simulink model "GRM_Airframe"  (R2018b)
settings: Solver=FixedStepAuto  StartTime=0.0  StopTime=T_sim  FixedStep=0.001  RelTol=1e-3
PreLoadFcn:
  | addpath('init_functions');
  | init_grm;
  | addpath('parameters');
  | para_def_grm;
values from neighbouring files (symbols this model uses):
  act_dmp = 0.6322    [para_def_grm.m]
  act_omega = 59.9250    (= 59.925)    [para_def_grm.m]
  aero = load('aero.mat')    [para_def_grm.m]
  c_be = -6.5e-3    (= -0.0065)    [init_grm.m]
  c_h_geop0 = 0    [init_grm.m]
  c_h_geope = 11e3    (= 11000)    [init_grm.m]
  c_pa0 = 101325    [init_grm.m]
  c_pe = -c_g0/c_be/sgc    (= 5.25587981272)    [init_grm.m]
  c_r0 = 6371000.79    [init_grm.m]
  c_rot = 7.292115e-5    (= 7.292115e-05)    [init_grm.m]
  c_Tmp0 = 288.15    [init_grm.m]
  d_siB_0 = 0    [para_def_grm.m]
  d_siB_max = deg2rad(1200)    [para_def_grm.m]
  d_siB_min = deg2rad(-1200)    [para_def_grm.m]
  dd_siB_max = deg2rad(50000)    [para_def_grm.m]
  dd_siB_min = deg2rad(-50000)    [para_def_grm.m]
  de_JBBB_xx = JBBB_xx_0 - JBBB_xx_e    (= 0)    [para_def_grm.m]
  de_JBBB_yy = JBBB_yy_0 - JBBB_yy_e    (= 0)    [para_def_grm.m]
  de_JBBB_zz = JBBB_zz_0 - JBBB_zz_e    (= 0)    [para_def_grm.m]
  de_mM = m_fuel_lookup(end)    [para_def_grm.m]
  F_prp = [450.52;428.7;423.25;391.61;352.34;304.35;266.17;243.26;216.92 ... (first row only)    [para_def_grm.m]
  flag_I_aero_switch = 1    [init_grm.m]
  flag_I_flat = 1    [init_grm.m]
  flag_I_gravity_switch = 1    [init_grm.m]
  flag_I_rot = 0    [init_grm.m]
  hcr = 1.4    [init_grm.m]
  J0PB_e = TBP*J0PP_e*TBP'    [para_def_grm.m]
  JMMM_0 = TBP*J0PP_0*TBP'    [para_def_grm.m]
  JMMM_e = TBP*J0PP_e*TBP'    [para_def_grm.m]
  lat_0 = 0    [init_grm.m]
  lon_0 = 0    [init_grm.m]
  m0 = mB_0    (= 3.30977)    [para_def_grm.m]
  m_fuel_lookup = [0;0.0573;0.1127;0.1667;0.2186;0.2681;0.3149;0.3588 ... (first row only)    [para_def_grm.m]
  mB_0 = 3.30977    [para_def_grm.m]
  mM_0 = 1.119    [para_def_grm.m]
  mM_e = de_mM    [para_def_grm.m]
  p0PB = [x0PB;y0PB;z0PB]    [para_def_grm.m]
  pBII_0 = TIE_0*pBEE_0    [init_grm.m]
  pMPB = [xMPB;yMPB;zMPB]    [para_def_grm.m]
  pNPB = [0;0;0]    [para_def_grm.m]
  qEG_0 = q12_from_T12(TEG)    [init_grm.m]
  qIB_0 = qumul(qIG_0,qGB_0)    [init_grm.m]
  qIE_0 = q12_from_T12(TIE_0)    [init_grm.m]
  sgc = 287.05287    [init_grm.m]
  siB_0 = 0    [para_def_grm.m]
  siB_max = deg2rad(30)    [para_def_grm.m]
  siB_min = deg2rad(-30)    [para_def_grm.m]
  t_prp1 = [0.04;0.28;0.54;1;1.48;1.99;2.51;3;3.5;3.67;3.82;4]    [para_def_grm.m]
  t_prp2 = t_prp2'    [para_def_grm.m]
  Tr3r4 = [1,1,1,1;1,1,-1,-1;-1,1,1,-1]*0.25    [para_def_grm.m]
  tRRR = 0    [para_def_grm.m]
  unc_act_bl = 0    [para_def_grm.m]
  unc_act_off = 0    [para_def_grm.m]
  unc_act_scale = 1    [para_def_grm.m]
  unc_aero_Cl_scale = 1    [para_def_grm.m]
  unc_aero_Cm_scale = 1    [para_def_grm.m]
  unc_aero_Cn_scale = 1    [para_def_grm.m]
  unc_aero_Cx_scale = 1    [para_def_grm.m]
  unc_aero_Cy_scale = 1    [para_def_grm.m]
  unc_aero_Cz_scale = 1    [para_def_grm.m]
  unc_cg_x = 0    [para_def_grm.m]
  unc_cg_y = 0    [para_def_grm.m]
  unc_cg_z = 0    [para_def_grm.m]
  unc_mB_bl = 0    [para_def_grm.m]
  unc_mB_scale = 1    [para_def_grm.m]
  unc_moi_Jxx = 0    [para_def_grm.m]
  unc_moi_Jyy = 0    [para_def_grm.m]
  unc_moi_Jzz = 0    [para_def_grm.m]
  unc_prp_scale = 1    [para_def_grm.m]
  unc_prp_x = 0    [para_def_grm.m]
  unc_prp_y = 0    [para_def_grm.m]
  unc_prp_z = 0    [para_def_grm.m]
  vBII_0 = vBEE_0 + cross(wIEI_0,pBII_0)    [init_grm.m]
  wBIB_0 = r2_from_r1_trans_q21(wBII_0,qBI_0)    [init_grm.m]
  x0PB = -0.5    [para_def_grm.m]
  xMPB = -0.9    [para_def_grm.m]
  y0PB = 0    [para_def_grm.m]
  yMPB = 0    [para_def_grm.m]
  z0PB = 0    [para_def_grm.m]
  zMPB = 0    [para_def_grm.m]
undefined symbols (not defined in the file or in its folder): c_b_WGS, c_flat, c_grav, c_rsma, d_mB_lookup, t_dmB
libraries: simulink_extras x11, simulink x3
(part 2 of 6)

== system GRM_Airframe/GRM_Airframe/weight_and_balance/d_moi ==
  prp : Inport
  Bus Selector1 : BusSelector  OutputSignals=dmB
  Constant : Constant  Value=de_JBBB_zz
  Constant1 : Constant  Value=de_JBBB_xx
  Constant2 : Constant  Value=de_JBBB_yy
  Constant5 : Constant  Value=de_mM
  Divide : Product  Inputs=*/
  Divide1 : Product  Inputs=*/
  Divide2 : Product  Inputs=*/
  Product : Product
  Vector Concatenate : Concatenate  NumInputs=3
  vector2diagonal_matrix : Subsystem
  d_JBBB : Outport
  wires:
  Constant2/1 -> Divide1/1
  prp/1 -> Bus Selector1/1
  Vector Concatenate/1 -> vector2diagonal_matrix/1(vector)
  Constant1/1 -> Divide2/1
  Divide/1 -> Vector Concatenate/3
  Divide1/1 -> Vector Concatenate/2
  Constant/1 -> Divide/1
  Constant5/1 -> Divide/2, Divide1/2, Divide2/2
  Divide2/1 -> Vector Concatenate/1
  Bus Selector1/1 -> Product/2  "<dmB>"
  vector2diagonal_matrix/1(diagonal_matrix) -> Product/1
  Product/1 -> d_JBBB/1  "d_JBBB"

== system GRM_Airframe/GRM_Airframe/weight_and_balance/mass ==
  sim_time_launch : Inport
  1-D Lookup Table : Lookup_n-D  NumberOfTableDimensions=1  BreakpointsForDimension1=t_prp2  Table=m_fuel_lookup  ExtrapMethod=Clip  DiagnosticForOutOfRangeInput=Warning  UseLastTableValue=on  InternalRulePriority=Speed  RndMeth=Simplest  InputSameDT=on
  Add : Sum  Inputs=+-
  Constant : Constant  Value=0
  Constant1 : Constant  Value=mB_0
  Constant2 : Constant  Value=mM_0
  Saturation : Saturate  UpperLimit=t_prp2(end)  LowerLimit=0
      settings: AttributesFormatString=|
      | %<UpperLimit>
      | %<LowerLimit>
  Subtract1 : Sum  Inputs=+-+
  Switch : Switch  Criteria=u2 > Threshold
  Switch1 : Switch  Criteria=u2 > Threshold
  mB_c : Outport
  mM : Outport  Port=2
  wires:
  Add/1 -> mM/1  "mM"
  Constant2/1 -> Add/1, Subtract1/3
  Saturation/1 -> 1-D Lookup Table/1
  sim_time_launch/1 -> Switch/2, Switch/1
  Constant/1 -> Switch/3
  1-D Lookup Table/1 -> Switch1/1
  Switch/1 -> Switch1/3, Switch1/2, Saturation/1
  Subtract1/1 -> mB_c/1  "mB_c"
  Switch1/1 -> Subtract1/2, Add/2
  Constant1/1 -> Subtract1/1

== system GRM_Airframe/GRM_Airframe/weight_and_balance/mass_uncertainty ==
  mB_c : Inport
  Add : Sum
  Constant : Constant  Value=unc_mB_bl
  Constant1 : Constant  Value=unc_mB_scale
  Product : Product
  mB : Outport
  wires:
  Product/1 -> Add/2
  Constant1/1 -> Product/2
  Add/1 -> mB/1  "mB"
  mB_c/1 -> Product/1
  Constant/1 -> Add/1

== system GRM_Airframe/GRM_Airframe/weight_and_balance/moi ==
  pBPB : Inport
  mM : Inport  Port=2
  Add : Sum
  Add4 : Sum
  Add5 : Sum
  Constant15 : Constant  Value=J0PB_e
  JMMM_linear_interpolation : Subsystem
  moi_coordinate_transformation : Subsystem
  moi_uncertainty : Subsystem
  steiners_theorem_missile : Subsystem
  steiners_theorem_motor : Subsystem
  JBBB : Outport
  wires:
  moi_uncertainty/1(JBBB) -> JBBB/1
  Add4/1 -> moi_uncertainty/1(JBBB_c)  "JBBB_c"
  steiners_theorem_missile/1(J_deviation) -> Add5/2
  Add5/1 -> Add4/1  "J0BB"
  Constant15/1 -> Add5/1
  Add/1 -> Add4/2  "JMBB"
  steiners_theorem_motor/1(JM_deviation) -> Add/1
  pBPB/1 -> steiners_theorem_motor/1(pBPB), steiners_theorem_missile/1(pBPB)
  moi_coordinate_transformation/1(JMMB) -> Add/2
  JMMM_linear_interpolation/1(JMMM) -> moi_coordinate_transformation/1(JMMM)
  mM/1 -> JMMM_linear_interpolation/1(mM), steiners_theorem_motor/2(mM)

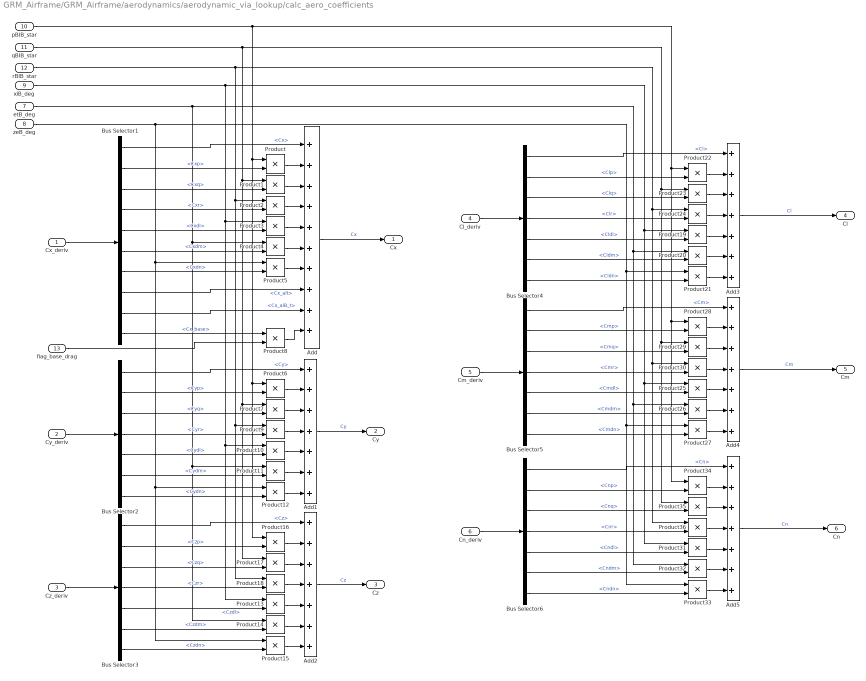
== system GRM_Airframe/GRM_Airframe/aerodynamics/aerodynamic_via_lookup/calc_aero_coefficients ==
  Cx_deriv : Inport
  Cy_deriv : Inport  Port=2
  Cz_deriv : Inport  Port=3
  Cl_deriv : Inport  Port=4
  Cm_deriv : Inport  Port=5
  Cn_deriv : Inport  Port=6
  etB_deg : Inport  Port=7
  zeB_deg : Inport  Port=8
  xiB_deg : Inport  Port=9
  pBIB_star : Inport  Port=10
  qBIB_star : Inport  Port=11
  rBIB_star : Inport  Port=12
  flag_base_drag : Inport  Port=13
  Add : Sum  Inputs=++++++++++
  Add{1..5} (5 alike) : Sum  Inputs=+++++++
  Bus Selector1 : BusSelector  OutputSignals=Cx,Cxp,Cxq,Cxr,Cxdl,Cxdm,Cxdn,Cx_alt,Cx_alB_t,Cx_base
  Bus Selector2 : BusSelector  OutputSignals=Cy,Cyp,Cyq,Cyr,Cydl,Cydm,Cydn
  Bus Selector3 : BusSelector  OutputSignals=Cz,Czp,Czq,Czr,Czdl,Czdm,Czdn
  Bus Selector4 : BusSelector  OutputSignals=Cl,Clp,Clq,Clr,Cldl,Cldm,Cldn
  Bus Selector5 : BusSelector  OutputSignals=Cm,Cmp,Cmq,Cmr,Cmdl,Cmdm,Cmdn
  Bus Selector6 : BusSelector  OutputSignals=Cn,Cnp,Cnq,Cnr,Cndl,Cndm,Cndn
  Product{,1..36} (37 alike) : Product
  Cx : Outport
  Cy : Outport  Port=2
  Cz : Outport  Port=3
  Cl : Outport  Port=4
  Cm : Outport  Port=5
  Cn : Outport  Port=6
  wires:
  zeB_deg/1 -> Product5/1, Product12/1, Product15/1, Product21/1, Product33/1, Product27/1
  Bus Selector6/1 -> Add5/1  "<Cn>"
  Bus Selector6/7 -> Product33/2  "<Cndn>"
  Bus Selector6/6 -> Product32/2  "<Cndm>"
  Bus Selector6/5 -> Product31/2  "<Cndl>"
  Bus Selector6/4 -> Product36/2  "<Cnr>"
  Bus Selector6/3 -> Product35/2  "<Cnq>"
  Bus Selector6/2 -> Product34/2  "<Cnp>"
  Add5/1 -> Cn/1  "Cn"
  Product33/1 -> Add5/7
  Product32/1 -> Add5/6
  Product31/1 -> Add5/5
  Product36/1 -> Add5/4
  Product35/1 -> Add5/3
  Product34/1 -> Add5/2
  Bus Selector5/7 -> Product27/2  "<Cmdn>"
  Bus Selector5/6 -> Product26/2  "<Cmdm>"
  Bus Selector5/5 -> Product25/2  "<Cmdl>"
  Bus Selector5/4 -> Product30/2  "<Cmr>"
  Bus Selector5/3 -> Product29/2  "<Cmq>"
  Bus Selector5/2 -> Product28/2  "<Cmp>"
  Bus Selector5/1 -> Add4/1  "<Cm>"
  Add4/1 -> Cm/1  "Cm"
  Product27/1 -> Add4/7
  Product26/1 -> Add4/6
  Product25/1 -> Add4/5
  Product30/1 -> Add4/4
  Product29/1 -> Add4/3
  Product28/1 -> Add4/2
  Bus Selector4/1 -> Add3/1  "<Cl>"
  Bus Selector4/7 -> Product21/2  "<Cldn>"
  Bus Selector4/6 -> Product20/2  "<Cldm>"
  Bus Selector4/5 -> Product19/2  "<Cldl>"
  Bus Selector4/4 -> Product24/2  "<Clr>"
  Bus Selector4/3 -> Product23/2  "<Clq>"
  Bus Selector4/2 -> Product22/2  "<Clp>"
  Add3/1 -> Cl/1  "Cl"
  Product21/1 -> Add3/7
  Product20/1 -> Add3/6
  Product19/1 -> Add3/5
  Product24/1 -> Add3/4
  Product23/1 -> Add3/3
  Product22/1 -> Add3/2
  Bus Selector3/7 -> Product15/2  "<Czdn>"
  Bus Selector3/6 -> Product14/2  "<Czdm>"
  Bus Selector3/5 -> Product13/2  "<Czdl>"
  Bus Selector3/4 -> Product18/2  "<Czr>"
  Bus Selector3/3 -> Product17/2  "<Czq>"
  Bus Selector3/1 -> Add2/1  "<Cz>"
  Bus Selector3/2 -> Product16/2  "<Czp>"
  Add2/1 -> Cz/1  "Cz"
  Product15/1 -> Add2/7
  Product14/1 -> Add2/6
  Product13/1 -> Add2/5
  Product18/1 -> Add2/4
  Product17/1 -> Add2/3
  Product16/1 -> Add2/2
  Add1/1 -> Cy/1  "Cy"
  Add/1 -> Cx/1  "Cx"
  rBIB_star/1 -> Product2/1, Product9/1, Product18/1, Product24/1, Product30/1, Product36/1
  qBIB_star/1 -> Product1/1, Product7/1, Product17/1, Product23/1, Product29/1, Product35/1
  pBIB_star/1 -> Product/1, Product6/1, Product16/1, Product22/1, Product28/1, Product34/1
  Bus Selector2/7 -> Product12/2  "<Cydn>"
  Bus Selector2/6 -> Product11/2  "<Cydm>"
  Bus Selector2/5 -> Product10/2  "<Cydl>"
  Bus Selector2/4 -> Product9/2  "<Cyr>"
  Bus Selector2/3 -> Product7/2  "<Cyq>"
  Product12/1 -> Add1/7
  Product11/1 -> Add1/6
  Product10/1 -> Add1/5
  Product9/1 -> Add1/4
  Product7/1 -> Add1/3
  Bus Selector2/2 -> Product6/2  "<Cyp>"
  Product6/1 -> Add1/2
  Bus Selector2/1 -> Add1/1  "<Cy>"
  etB_deg/1 -> Product4/1, Product11/1, Product14/1, Product20/1, Product26/1, Product32/1
  xiB_deg/1 -> Product3/1, Product10/1, Product13/1, Product19/1, Product25/1, Product31/1
  flag_base_drag/1 -> Product8/2
  Bus Selector1/10 -> Product8/1  "<Cx_base>"
  Product8/1 -> Add/10
  Bus Selector1/9 -> Add/9  "<Cx_alB_t>"
  Bus Selector1/8 -> Add/8  "<Cx_alt>"
  Product5/1 -> Add/7
  Bus Selector1/7 -> Product5/2  "<Cxdn>"
  Product4/1 -> Add/6
  Bus Selector1/6 -> Product4/2  "<Cxdm>"
  Product3/1 -> Add/5
  Bus Selector1/5 -> Product3/2  "<Cxdl>"
  Product2/1 -> Add/4
  Bus Selector1/4 -> Product2/2  "<Cxr>"
  Bus Selector1/3 -> Product1/2  "<Cxq>"
  Product1/1 -> Add/3
  Product/1 -> Add/2
  Bus Selector1/2 -> Product/2  "<Cxp>"
  Bus Selector1/1 -> Add/1  "<Cx>"
  Cl_deriv/1 -> Bus Selector4/1
  Cz_deriv/1 -> Bus Selector3/1
  Cm_deriv/1 -> Bus Selector5/1
  Cn_deriv/1 -> Bus Selector6/1
  Cy_deriv/1 -> Bus Selector2/1
  Cx_deriv/1 -> Bus Selector1/1

== system GRM_Airframe/GRM_Airframe/aerodynamics/aerodynamic_via_lookup/calc_aero_for_mom ==
  hBE : Inport
  pBSB : Inport  Port=2
  qdynB : Inport  Port=3
  Cx : Inport  Port=4
  Cy : Inport  Port=5
  Cz : Inport  Port=6
  Cl : Inport  Port=7
  Cm : Inport  Port=8
  Cn : Inport  Port=9
  Add : Sum
  Constant1 : Constant  Value=aero.lref
  Constant2 : Constant  Value=aero.sref
  Product : Product
  Product1 : Product  Inputs=3
  Product2 : Product
  Vector Concatenate1 : Concatenate  NumInputs=3
  Vector Concatenate2 : Concatenate  NumInputs=3
  cross_product : Subsystem
      mask help: cross product r3 = r1 x r2
      mask Help:
      | Name:
      | 
      |     cross_product
      | 
      | Description:
      | 
      |     This block implements the cross product r3 = r1 x r2.
      | 
      | Inputs  [size] [data type] [unit]:
      | 
      |     vector 1  [3] [double] [-]
      |     vector 2  [3] [double] [-]
      | 
      | Outputs  [size] [data type] [unit]:
      | 
      |     resulting vector  [3] [double] [-]
      mask Display: disp(' r3 = r1 x r2')
  launch_rail : Subsystem
  launch_rail1 : Subsystem
  FBAB : Outport
  MBAB : Outport  Port=2
  wires:
  launch_rail/1(FBAB) -> FBAB/1
  launch_rail1/1(MBAB) -> MBAB/1
  hBE/1 -> launch_rail/1(hBE), launch_rail1/1(hBE)
  cross_product/1(r1_x_r2) -> Add/1
  Product2/1 -> Product/2, Product1/1
  Constant2/1 -> Product2/1
  Constant1/1 -> Product1/3
  Add/1 -> launch_rail1/2(MBAB_c)  "MBAB"
  Product1/1 -> Add/2  "MBAB"
  Product/1 -> cross_product/2(r2), launch_rail/2(FBAB_c)  "FBAB"
  pBSB/1 -> cross_product/1(r1)
  Vector Concatenate2/1 -> Product/1
  Vector Concatenate1/1 -> Product1/2
  qdynB/1 -> Product2/2
  Cn/1 -> Vector Concatenate1/3
  Cl/1 -> Vector Concatenate1/1
  Cx/1 -> Vector Concatenate2/1
  Cz/1 -> Vector Concatenate2/3
  Cm/1 -> Vector Concatenate1/2
  Cy/1 -> Vector Concatenate2/2

== system GRM_Airframe/GRM_Airframe/aerodynamics/aerodynamic_via_lookup/calc_derivatives ==
  hBE : Inport
  MaB : Inport  Port=2
  alB : Inport  Port=3
  beB : Inport  Port=4
  etB_deg : Inport  Port=5
  zeB_deg : Inport  Port=6
  Cl_derivatives_lookup : Subsystem
  Cm_derivatives_lookup : Subsystem
  Cn_derivatives_lookup : Subsystem
  Cx_derivatives_lookup : Subsystem
  Cy_derivatives_lookup : Subsystem
  Cz_derivatives_lookup : Subsystem
  aerodynamics_pre_lookup : Subsystem
  calc_total_deflection_angle : Subsystem
  Cx_deriv : Outport
  Cy_deriv : Outport  Port=2
  Cz_deriv : Outport  Port=3
  Cl_deriv : Outport  Port=4
  Cm_deriv : Outport  Port=5
  Cn_deriv : Outport  Port=6
  wires:
  zeB_deg/1 -> calc_total_deflection_angle/2(zeB_deg)
  etB_deg/1 -> calc_total_deflection_angle/1(etB_deg)
  beB/1 -> aerodynamics_pre_lookup/2(beB), calc_total_deflection_angle/4(beB)
  alB/1 -> aerodynamics_pre_lookup/1(alB), calc_total_deflection_angle/3(alB)
  calc_total_deflection_angle/1(delta_t) -> Cx_derivatives_lookup/1(delta_t)
  hBE/1 -> Cx_derivatives_lookup/2(hBE)
  aerodynamics_pre_lookup/1(aero_pre_lookup) -> Cx_derivatives_lookup/3(aero_pre_lookup), Cy_derivatives_lookup/1(aero_pre_lookup), Cz_derivatives_lookup/1(aero_pre_lookup), Cl_derivatives_lookup/1(aero_pre_lookup), Cm_derivatives_lookup/1(aero_pre_lookup), Cn_derivatives_lookup/1(aero_pre_lookup)
  Cl_derivatives_lookup/1(Cl_deriv) -> Cl_deriv/1
  Cm_derivatives_lookup/1(Cm_deriv) -> Cm_deriv/1
  Cz_derivatives_lookup/1(Cz_deriv) -> Cz_deriv/1
  Cy_derivatives_lookup/1(Cy_deriv) -> Cy_deriv/1
  MaB/1 -> aerodynamics_pre_lookup/3(Ma)
  Cx_derivatives_lookup/1(Cx_deriv) -> Cx_deriv/1
  Cn_derivatives_lookup/1(Cn_deriv) -> Cn_deriv/1

== system GRM_Airframe/GRM_Airframe/aerodynamics/aerodynamic_via_lookup/transform_rad2deg_al_be ==
  alB : Inport
  beB : Inport  Port=2
  Radians to Degrees : simulink_extras/Transformations/Radians to Degrees
  Radians to Degrees1 : simulink_extras/Transformations/Radians to Degrees
  alB_deg : Outport
  beB_deg : Outport  Port=2
  wires:
  beB/1 -> Radians to Degrees1/1
  Radians to Degrees1/1 -> beB_deg/1  "beB_deg"
  Radians to Degrees/1 -> alB_deg/1  "alB_deg"
  alB/1 -> Radians to Degrees/1

== system GRM_Airframe/GRM_Airframe/aerodynamics/aerodynamic_via_lookup/transform_rad2deg_fin ==
  afinB : Inport
  Demux : Demux  Outputs=3
  Radians to Degrees : simulink_extras/Transformations/Radians to Degrees
  Radians to Degrees1 : simulink_extras/Transformations/Radians to Degrees
  Radians to Degrees2 : simulink_extras/Transformations/Radians to Degrees
  etB_deg : Outport
  zeB_deg : Outport  Port=2
  xiB_deg : Outport  Port=3
  wires:
  Demux/1 -> Radians to Degrees/1  "xiB"
  afinB/1 -> Demux/1
  Demux/3 -> Radians to Degrees2/1  "zeB"
  Demux/2 -> Radians to Degrees1/1  "etB"
  Radians to Degrees1/1 -> etB_deg/1  "etB_deg"
  Radians to Degrees2/1 -> zeB_deg/1  "zeB_deg"
  Radians to Degrees/1 -> xiB_deg/1  "xiB_deg"

== system GRM_Airframe/GRM_Airframe/aerodynamics/aerodynamic_via_lookup/transform_rad2deg_rates ==
  wBIB_star : Inport
  Demux : Demux  Outputs=3
  Radians to Degrees : simulink_extras/Transformations/Radians to Degrees
  Radians to Degrees1 : simulink_extras/Transformations/Radians to Degrees
  Radians to Degrees2 : simulink_extras/Transformations/Radians to Degrees
  pBIB_star_deg : Outport
  qBIB_star_deg : Outport  Port=2
  rBIB_star_deg : Outport  Port=3
  wires:
  Radians to Degrees1/1 -> qBIB_star_deg/1  "qBIB_star_deg"
  Demux/2 -> Radians to Degrees1/1
  Radians to Degrees/1 -> pBIB_star_deg/1  "pBIB_star_deg"
  Demux/1 -> Radians to Degrees/1
  wBIB_star/1 -> Demux/1
  Radians to Degrees2/1 -> rBIB_star_deg/1  "rBIB_star_deg"
  Demux/3 -> Radians to Degrees2/1

== system GRM_Airframe/GRM_Airframe/environment/WGS84_Gravitation/WGS84_2_ECEF ==
  h : Inport
  lon : Inport  Port=2
  lat : Inport  Port=3
  Add1 : Sum  Inputs=+-
  Add2 : Sum
  Add3 : Sum
  Constant : Constant
  Divide : Product  Inputs=***
  Divide1 : Product  Inputs=***
  Divide2 : Product  Inputs=**
  Divide3 : Product  Inputs=**
  Divide4 : Product  Inputs=**
  Mux : Mux  Inputs=3
  Trigonometric Function : Trigonometry
  Trigonometric Function1 : Trigonometry  Operator=cos
  Trigonometric Function2 : Trigonometry
  Trigonometric Function3 : Trigonometry  Operator=cos
  "WGS84 Transformation Parameter " : Subsystem
  pE : Outport
  wires:
  Trigonometric Function/1 -> Divide1/2  "sin(lambda)"
  Trigonometric Function2/1 -> Divide4/2  "sin(phi)"
  Add3/1 -> Divide/1, Divide1/1
  lon/1 -> Trigonometric Function/1, Trigonometric Function1/1
  Mux/1 -> pE/1  "pE"
  Trigonometric Function3/1 -> Divide/3, Divide1/3  "cos(phi)"
  Trigonometric Function1/1 -> Divide/2  "cos(lambda)"
  h/1 -> Add3/1, Add2/1
  "WGS84 Transformation Parameter "/2(e) -> Divide2/1, Divide2/2
  "WGS84 Transformation Parameter "/1(N) -> Divide3/1, Add3/2
  Divide4/1 -> Mux/3  "z_ECEF"
  Add1/1 -> Divide3/2
  Constant/1 -> Add1/1
  Divide3/1 -> Add2/2  "N(1-e^2)"
  Divide2/1 -> Add1/2
  lat/1 -> Trigonometric Function2/1, Trigonometric Function3/1, "WGS84 Transformation Parameter "/1(phi)
  Divide/1 -> Mux/1  "x_ECEF"
  Add2/1 -> Divide4/1
  Divide1/1 -> Mux/2  "y_ECEF"

== system GRM_Airframe/GRM_Airframe/environment/atmosphere_static_ISO_2533/density ==
  Tmp : Inport
  pa : Inport  Port=2
  Divide : Product  Inputs=/*/
  specific_gas_constant : Constant  Value=sgc
  rho : Outport
  wires:
  specific_gas_constant/1 -> Divide/3
  pa/1 -> Divide/2
  Divide/1 -> rho/1  "rho"
  Tmp/1 -> Divide/1

== system GRM_Airframe/GRM_Airframe/environment/atmosphere_static_ISO_2533/geopot_height ==
  hBE : Inport
  Add : Sum
  Divide : Product  Inputs=*/*
  mean_earth_radius : Constant  Value=mean_earth_radius
  h_geop : Outport
  wires:
  Add/1 -> Divide/2
  hBE/1 -> Divide/1, Add/1
  Divide/1 -> h_geop/1  "h_geop"
  mean_earth_radius/1 -> Add/2, Divide/3

== system GRM_Airframe/GRM_Airframe/environment/atmosphere_static_ISO_2533/speed_of_sound ==
  Tmp : Inport
  Product : Product  Inputs=3
  Sqrt : Sqrt  SaturateOnIntegerOverflow=on
  heat_capacity_ratio : Constant  Value=hcr
  specific_gas_constant : Constant  Value=sgc
  sos : Outport
  wires:
  specific_gas_constant/1 -> Product/1
  heat_capacity_ratio/1 -> Product/2
  Product/1 -> Sqrt/1
  Tmp/1 -> Product/3
  Sqrt/1 -> sos/1  "sos"

== system GRM_Airframe/GRM_Airframe/environment/atmosphere_static_ISO_2533/tmp_and_pressure_ISO_2533 ==
  h_geop : Inport
  e_Tmp : Inport  Port=2
  e_pa : Inport  Port=3
  Subtract1 : Sum
  Subtract2 : Sum
  Tmp_norm_msl : Constant  Value=c_Tmp0
  geopotential_height_ref : Constant  Value=c_h_geop0
  pa_norm_msl : Constant  Value=c_pa0
  static_Temperature : Subsystem
  static_pressure : Subsystem
  Tmp : Outport
  pa : Outport  Port=2
  wires:
  Tmp_norm_msl/1 -> Subtract1/2
  geopotential_height_ref/1 -> static_Temperature/3(h_geop_ref), static_pressure/1(h_geop_ref)  "h_geop_ref"
  e_Tmp/1 -> Subtract1/1
  static_Temperature/1(Tmp) -> Tmp/1
  e_pa/1 -> Subtract2/1
  static_pressure/1(pa) -> pa/1
  Subtract1/1 -> static_Temperature/1(Tmp_ref), static_pressure/3(Tmp_ref)  "Tmp_ref"
  pa_norm_msl/1 -> Subtract2/2
  Subtract2/1 -> static_pressure/4(pa_ref)  "pa_ref"
  h_geop/1 -> static_Temperature/2(h_geop), static_pressure/2(h_geop)

== system GRM_Airframe/GRM_Airframe/gravity/launch_rail/initial_altitude ==
  Constant : Constant  Value=pBII_0
  Constant2 : Constant  Value=flag_I_flat
  Demux : Demux  Outputs=3
  Gain : Gain  Gain=-1
  Switch1 : Switch  Criteria=u2 > Threshold
  Terminator{,1..3} (4 alike) : Terminator
  trafo_E_to_geodetic : Subsystem  mask(Transformation der ECEF Position in geodätische Größen){}
      mask help: Dieser Block transformiert die Position im ECEF KOS in die geodätische Länge, Breite und Höhe
      mask init:
      | [c_mue, c_rsma, c_flat] = init_transformations_earth;
      mask Help:
      | Name:
      | 
      |     trafo_E_to_geodetic
      | 
      | Beschreibung:
      | 
      |     Dieser Block transformiert die Position im ECEF KOS in die geodätische
      |     Länge, Breite und Höhe.
      | 
      | Inputs   [size]  [data type] [unit]:
      | 
      |     pBEE    [3] [double] [m]
      | 
      | Outputs  [size]  [data type] [unit]:
      | 
      |     long  [1] [double] [rad]
      |     lat   [1] [double] [rad]
      |     alt   [1] [double] [m]
      | 
      | Parameter
      | 
      |    c_rsma
      |    c_flat
  hBE_0 : Outport
  wires:
  Switch1/1 -> hBE_0/1  "hBE_0"
  trafo_E_to_geodetic/1(lon) -> Terminator/1
  Constant/1 -> trafo_E_to_geodetic/1(pBEE), Demux/1
  trafo_E_to_geodetic/2(lat) -> Terminator1/1
  Demux/1 -> Terminator2/1
  Gain/1 -> Switch1/1
  Demux/3 -> Gain/1
  Demux/2 -> Terminator3/1
  trafo_E_to_geodetic/3(alt) -> Switch1/3  "hBE_0"
  Constant2/1 -> Switch1/2

== system GRM_Airframe/GRM_Airframe/motion_kinematics/calc_motion_kinematics/calc_transformation_matrix ==
  qIE : Inport
  qEG : Inport  Port=2
  qIB : Inport  Port=3
  T12_from_q1 : Subsystem
      mask help: Transforms a quaternion into a Direction Cosine Matrix
      mask Help:
      | Name:
      | 
      |     T12_from_q12
      | 
      | Description:
      | 
      |     This block implements the transformation of a quaternion into the
      |     corresponding direction cosine matrix DCM.
      | 
      | Inputs  [size] [data type] [unit]:
      | 
      |     quaternion q12 [4] [double] [-]
      | 
      | Outputs  [size] [data type] [unit]:
      | 
      |     direction cosine matrix T12  [3x3] [double] [-]
      mask Display:
      | %port_label('input', 1, 'q12')
      | %port_label('output', 1, 'T12')
      | disp('q \rightarrow DCM','texmode','on')
  T12_from_q12 : Subsystem
      mask help: Transforms a quaternion into a Direction Cosine Matrix
      mask Help:
      | Name:
      | 
      |     T12_from_q12
      | 
      | Description:
      | 
      |     This block implements the transformation of a quaternion into the
      |     corresponding direction cosine matrix DCM.
      | 
      | Inputs  [size] [data type] [unit]:
      | 
      |     quaternion q12 [4] [double] [-]
      | 
      | Outputs  [size] [data type] [unit]:
      | 
      |     direction cosine matrix T12  [3x3] [double] [-]
      mask Display:
      | %port_label('input', 1, 'q12')
      | %port_label('output', 1, 'T12')
      | disp('q \rightarrow DCM','texmode','on')
  T12_from_q2 : Subsystem
      mask help: Transforms a quaternion into a Direction Cosine Matrix
      mask Help:
      | Name:
      | 
      |     T12_from_q12
      | 
      | Description:
      | 
      |     This block implements the transformation of a quaternion into the
      |     corresponding direction cosine matrix DCM.
      | 
      | Inputs  [size] [data type] [unit]:
      | 
      |     quaternion q12 [4] [double] [-]
      | 
      | Outputs  [size] [data type] [unit]:
      | 
      |     direction cosine matrix T12  [3x3] [double] [-]
      mask Display:
      | %port_label('input', 1, 'q12')
      | %port_label('output', 1, 'T12')
      | disp('q \rightarrow DCM','texmode','on')
  conjugate_quaternion : Subsystem
      mask help: conjugate a quaternion
      mask Help:
      | Name:
      | 
      |     conjugate_quaternion
      | 
      | Description:
      | 
      |     computes the conjugate quaternion
      | 
      | Inputs  [size] [data type] [unit]:
      | 
      |     quaternion q_2_1  [4] [double] [-]
      | 
      | Outputs  [size] [data type] [unit]:
      | 
      |     conjugated quaternion q_1_2  [4] [double] [-]
      mask Display: disp (' conj(q)')
  q31_from_q32_mul_q1 : Subsystem
      mask help: multiply two quaternions
      mask Help:
      | Name:
      | 
      |     q31_from_q32_mul_q21
      | 
      | Description:
      | 
      |     This block implements the multiplication of two quaternions according
      |     to q31=q32*q21.
      | 
      | Inputs  [size] [data type] [unit]:
      | 
      |     attitude quaternion q32  [4] [double] [-]
      |     attitude quaternion q21  [4] [double] [-]
      | 
      | Outputs  [size] [data type] [unit]:
      | 
      |     attitude quaternion q31  [4] [double] [-]
      mask Display:
      | port_label('input', 1, 'q32')
      | port_label('input', 2, 'q21')
      | port_label('output', 1, 'q31')
      | disp('q_{31} = q_{32} {\bf\cdot} q_{21}','texmode','on')
  q31_from_q32_mul_q2 : Subsystem
      mask help: multiply two quaternions
      mask Help:
      | Name:
      | 
      |     q31_from_q32_mul_q21
      | 
      | Description:
      | 
      |     This block implements the multiplication of two quaternions according
      |     to q31=q32*q21.
      | 
      | Inputs  [size] [data type] [unit]:
      | 
      |     attitude quaternion q32  [4] [double] [-]
      |     attitude quaternion q21  [4] [double] [-]
      | 
      | Outputs  [size] [data type] [unit]:
      | 
      |     attitude quaternion q31  [4] [double] [-]
      mask Display:
      | port_label('input', 1, 'q32')
      | port_label('input', 2, 'q21')
      | port_label('output', 1, 'q31')
      | disp('q_{31} = q_{32} {\bf\cdot} q_{21}','texmode','on')
  q31_from_q32_mul_q21 : Subsystem
      mask help: multiply two quaternions
      mask Help:
      | Name:
      | 
      |     q31_from_q32_mul_q21
      | 
      | Description:
      | 
      |     This block implements the multiplication of two quaternions according
      |     to q31=q32*q21.
      | 
      | Inputs  [size] [data type] [unit]:
      | 
      |     attitude quaternion q32  [4] [double] [-]
      |     attitude quaternion q21  [4] [double] [-]
      | 
      | Outputs  [size] [data type] [unit]:
      | 
      |     attitude quaternion q31  [4] [double] [-]
      mask Display:
      | port_label('input', 1, 'q32')
      | port_label('input', 2, 'q21')
      | port_label('output', 1, 'q31')
      | disp('q_{31} = q_{32} {\bf\cdot} q_{21}','texmode','on')
  TEB : Outport
  TGB : Outport  Port=2
  TIB : Outport  Port=3
  wires:
  T12_from_q12/1(T12) -> TIB/1  "TIB"
  q31_from_q32_mul_q2/1(q31) -> T12_from_q1/1(q12)  "qEB"
  qIE/1 -> q31_from_q32_mul_q21/1(q32)
  conjugate_quaternion/1(q_conj) -> q31_from_q32_mul_q1/1(q32)  "qGI"
  T12_from_q1/1(T12) -> TEB/1  "TEB"
  qEG/1 -> q31_from_q32_mul_q2/1(q32), q31_from_q32_mul_q21/2(q21)
  q31_from_q32_mul_q1/1(q31) -> q31_from_q32_mul_q2/2(q21), T12_from_q2/1(q12)  "qGB"
  qIB/1 -> T12_from_q12/1(q12), q31_from_q32_mul_q1/2(q21)
  q31_from_q32_mul_q21/1(q31) -> conjugate_quaternion/1(q)  "qIG"
  T12_from_q2/1(T12) -> TGB/1  "TGB"

== system GRM_Airframe/GRM_Airframe/motion_kinematics/calc_motion_kinematics/earth_rotation ==
  lat : Inport
  lon : Inport  Port=2
  Gain : Gain  Gain=-1
  Gain1 : Gain  Gain=-1
  earth_rotation_rate : Subsystem
  quaternion_integration : Subsystem
  quaternion_integration1 : Subsystem
  transport_rate : Subsystem
  wIEE : Outport
  TIE : Outport  Port=2
  qIE : Outport  Port=3
  qEG : Outport  Port=4
  TEG : Outport  Port=5
  wEGG : Outport  Port=6
  wires:
  quaternion_integration1/2(TEG) -> TEG/1
  quaternion_integration1/1(qEG) -> qEG/1
  Gain1/1 -> quaternion_integration1/1(wGEG)  "wGEG"
  transport_rate/1(wEGG) -> Gain1/1, wEGG/1
  lon/1 -> transport_rate/2(lon)
  lat/1 -> transport_rate/1(lat)
  quaternion_integration/2(TIE) -> TIE/1
  quaternion_integration/1(qIE) -> qIE/1
  Gain/1 -> quaternion_integration/1(wEIE)  "wEIE"
  earth_rotation_rate/1(wIEE) -> Gain/1, wIEE/1

== system GRM_Airframe/GRM_Airframe/propulsion/prp_uncertainty/3_rot_mat ==
  wi1 : Inport
  wi2 : Inport  Port=2
  wi3 : Inport  Port=3
  1. Rotation x-Achse : Subsystem
  1. Rotation y-Achse : Subsystem
  1. Rotation z-Achse : Subsystem
  2. Rotation x-Achse : Subsystem
  2. Rotation y-Achse : Subsystem
  2. Rotation z-Achse : Subsystem
  3. Rotation : Product  Inputs=***  Multiplication=Matrix(*)
  3. Rotation x-Achse : Subsystem
  3. Rotation y-Achse : Subsystem
  3. Rotation z-Achse : Subsystem
  Constant : Constant  Value=rot_1
  Constant1 : Constant  Value=rot_2
  Constant2 : Constant  Value=rot_3
  Multiport Switch : MultiPortSwitch
  Multiport Switch1 : MultiPortSwitch
  Multiport Switch2 : MultiPortSwitch
  T12 : Outport
  wires:
  3. Rotation x-Achse/1(3Rot_Matrix_x) -> Multiport Switch2/2
  3. Rotation y-Achse/1(3Rot_Matrix_y) -> Multiport Switch2/3
  2. Rotation z-Achse/1(2Rot_Matrix_z) -> Multiport Switch1/4
  2. Rotation y-Achse/1(2Rot_Matrix_y) -> Multiport Switch1/3
  2. Rotation x-Achse/1(2Rot_Matrix_x) -> Multiport Switch1/2
  3. Rotation/1 -> T12/1  "T12"
  Constant2/1 -> Multiport Switch2/1
  1. Rotation z-Achse/1(1Rot_Matrix_z) -> Multiport Switch/4
  1. Rotation y-Achse/1(1Rot_Matrix_y) -> Multiport Switch/3
  Constant1/1 -> Multiport Switch1/1
  1. Rotation x-Achse/1(1Rot_Matrix_x) -> Multiport Switch/2
  Constant/1 -> Multiport Switch/1
  3. Rotation z-Achse/1(3Rot_Matrix_z) -> Multiport Switch2/4
  wi2/1 -> 2. Rotation x-Achse/1(alpha2), 2. Rotation y-Achse/1(alpha2), 2. Rotation z-Achse/1(alpha2)
  wi1/1 -> 1. Rotation x-Achse/1(alpha1), 1. Rotation y-Achse/1(alpha1), 1. Rotation z-Achse/1(alpha1)
  wi3/1 -> 3. Rotation y-Achse/1(alpha3), 3. Rotation z-Achse/1(alpha3), 3. Rotation x-Achse/1(alpha3)
  Multiport Switch/1 -> 3. Rotation/3
  Multiport Switch1/1 -> 3. Rotation/2
  Multiport Switch2/1 -> 3. Rotation/1

== system GRM_Airframe/GRM_Airframe/propulsion/prp_uncertainty/cross_product ==
  note: Inputs [size]:
      |
      | r1 [3x1]
      | r2 [3x1]
  note: Outputs [size]:
      |
      | r1 x r2  [3x1]
  r1 : Inport
  r2 : Inport  Port=2
  Demux2 : Demux  Outputs=[1;1;1]
  Demux3 : Demux  Outputs=[1;1;1]
  Product{2..7} (6 alike) : Product  SaturateOnIntegerOverflow=on  RndMeth=Zero  InputSameDT=on  OutDataTypeStr=Inherit: Same as first input
  Sum : Sum  Inputs=+-  SaturateOnIntegerOverflow=on  InputSameDT=on  OutDataTypeStr=Inherit: Same as first input
  Sum1 : Sum  Inputs=+-  SaturateOnIntegerOverflow=on  InputSameDT=on  OutDataTypeStr=Inherit: Same as first input
  Sum2 : Sum  Inputs=+-  SaturateOnIntegerOverflow=on  InputSameDT=on  OutDataTypeStr=Inherit: Same as first input
  Vector Concatenate : Concatenate  NumInputs=3  Mode=Multidimensional array
  r1_x_r2 : Outport  PortDimensions=[3,1]
  wires:
  Vector Concatenate/1 -> r1_x_r2/1
  r2/1 -> Demux3/1
  r1/1 -> Demux2/1
  Sum2/1 -> Vector Concatenate/3
  Sum1/1 -> Vector Concatenate/2
  Sum/1 -> Vector Concatenate/1
  Product7/1 -> Sum2/2
  Product6/1 -> Sum2/1
  Product5/1 -> Sum1/2
  Product4/1 -> Sum1/1
  Product3/1 -> Sum/2
  Product2/1 -> Sum/1
  Demux2/1 -> Product5/1, Product6/1
  Demux3/1 -> Product4/2, Product7/2
  Demux2/3 -> Product4/1, Product3/1
  Demux3/2 -> Product3/2, Product6/2
  Demux3/3 -> Product2/2, Product5/2
  Demux2/2 -> Product7/1, Product2/1

== system GRM_Airframe/GRM_Airframe/rb_eom/calc_bus_flight_dyn_bus_entries/Subsystem2 ==
  TIE : Inport
  pBII : Inport  Port=2
  Constant : Constant  Value=lon_0
  Constant1 : Constant  Value=flag_I_flat
  Constant2 : Constant  Value=lat_0
  Demux : Demux  Outputs=3
  Demux1 : Demux  Outputs=3
  Gain : Gain  Gain=-1
  Math Function : Math  Operator=transpose  SaturateOnIntegerOverflow=on
  Product : Product  Multiplication=Matrix(*)
  Switch : Switch  Criteria=u2 > Threshold
  Terminator : Terminator
  Terminator1 : Terminator
  Vector Concatenate : Concatenate  NumInputs=3
  Vector Concatenate1 : Concatenate  NumInputs=3
  trafo_E_to_geodetic : Subsystem  mask(Transformation der ECEF Position in geodätische Größen){}
      mask help: Dieser Block transformiert die Position im ECEF KOS in die geodätische Länge, Breite und Höhe
      mask init:
      | [c_mue, c_rsma, c_flat] = init_transformations_earth;
      mask Help:
      | Name:
      | 
      |     trafo_E_to_geodetic
      | 
      | Beschreibung:
      | 
      |     Dieser Block transformiert die Position im ECEF KOS in die geodätische
      |     Länge, Breite und Höhe.
      | 
      | Inputs   [size]  [data type] [unit]:
      | 
      |     pBEE    [3] [double] [m]
      | 
      | Outputs  [size]  [data type] [unit]:
      | 
      |     long  [1] [double] [rad]
      |     lat   [1] [double] [rad]
      |     alt   [1] [double] [m]
      | 
      | Parameter
      | 
      |    c_rsma
      |    c_flat
  lon : Outport
  lat : Outport  Port=2
  hBE : Outport  Port=3
  wires:
  Math Function/1 -> Product/1  "TEI"
  TIE/1 -> Math Function/1
  Switch/1 -> Demux1/1
  Vector Concatenate1/1 -> Switch/1
  Constant1/1 -> Switch/2
  Vector Concatenate/1 -> Switch/3
  Constant2/1 -> Vector Concatenate1/2
  Constant/1 -> Vector Concatenate1/1
  Gain/1 -> Vector Concatenate1/3
  Demux/3 -> Gain/1
  Demux/2 -> Terminator1/1
  Demux/1 -> Terminator/1
  trafo_E_to_geodetic/3(alt) -> Vector Concatenate/3  "alt"
  trafo_E_to_geodetic/2(lat) -> Vector Concatenate/2  "lat"
  trafo_E_to_geodetic/1(lon) -> Vector Concatenate/1  "lon"
  Demux1/3 -> hBE/1  "hBE"
  Demux1/1 -> lon/1  "lon"
  Product/1 -> trafo_E_to_geodetic/1(pBEE)  "pBEE"
  pBII/1 -> Product/2, Demux/1
  Demux1/2 -> lat/1  "lat"

== system GRM_Airframe/GRM_Airframe/rb_eom/calc_bus_flight_dyn_bus_entries/quaternion_to_euler_angles ==
  note: Um numerische Probleme zu
      | vermeiden, wird hier eine Saturiierung
      | benutzt.
  note: Outputs [size]:
      |
      | roll angle [1]
      | pitch angle [1]
      | yaw angle [1]
  note: Inputs [size]:
      |
      | quaternion [4]
  q : Inport  PortDimensions=4
  Add : Sum
  Add1 : Sum  Inputs=+--
  Add2 : Sum  Inputs=+-
  Add3 : Sum
  Add4 : Sum  Inputs=+--
  Complex to Real-Imag : ComplexToRealImag  Output=Real
  Constant : Constant  Value=0.5
  Constant1 : Constant  Value=0.5
  Demux : Demux
  Gain : Gain  Gain=2
  Product{,1..9} (10 alike) : Product
  Saturation : Saturate  UpperLimit=1  LowerLimit=-1
      settings: AttributesFormatString=|
      | %<UpperLimit>
      | %<LowerLimit>
  Trigonometric Function : Trigonometry  Operator=atan2
  Trigonometric Function1 : Trigonometry  Operator=asin
  Trigonometric Function2 : Trigonometry  Operator=atan2
  Vector Concatenate : Concatenate  NumInputs=3
  eulx : Outport
  wires:
  Vector Concatenate/1 -> Complex to Real-Imag/1
  Complex to Real-Imag/1 -> eulx/1
  Trigonometric Function2/1 -> Vector Concatenate/3
  Trigonometric Function1/1 -> Vector Concatenate/2
  Trigonometric Function/1 -> Vector Concatenate/1
  Add/1 -> Trigonometric Function/1
  Product1/1 -> Add/2
  Product/1 -> Add/1
  Product3/1 -> Add1/3
  Product2/1 -> Add1/2
  Product5/1 -> Add2/2
  Product4/1 -> Add2/1
  Product7/1 -> Add3/2
  Product6/1 -> Add3/1
  Add3/1 -> Trigonometric Function2/1
  Add4/1 -> Trigonometric Function2/2
  Add2/1 -> Gain/1
  Add1/1 -> Trigonometric Function/2
  q/1 -> Demux/1
  Demux/4 -> Product7/2, Product4/2, Product/2  "4"
  Demux/1 -> Product2/2, Product2/1, Product/1, Product6/1, Product5/1  "1"
  Demux/2 -> Product4/1, Product3/2, Product3/1, Product1/1, Product8/2, Product8/1, Product6/2  "2"
  Constant/1 -> Add1/1
  Product9/1 -> Add4/3
  Product8/1 -> Add4/2
  Constant1/1 -> Add4/1
  Demux/3 -> Product9/2, Product9/1, Product7/1, Product1/2, Product5/2  "3"
  Gain/1 -> Saturation/1
  Saturation/1 -> Trigonometric Function1/1

== system GRM_Airframe/GRM_Airframe/rb_eom/eom_6dof/Rigid_Body_EOM_6_DOF ==
  FBTX : Inport  PortDimensions=[3,1]
  MBTB : Inport  Port=2  PortDimensions=[3,1]
  mB : Inport  Port=3  PortDimensions=[1]
  x0 : Inport  Port=4
  JBB : Inport  Port=5  PortDimensions=[3,3]
  d_JBB : Inport  Port=6  PortDimensions=[3,3]
  Bus Selector : BusSelector  OutputSignals=qIB,vBII,wBIB
  Constant : Constant  Value=flag_Kraft
  Integration : Subsystem
  Math Function2 : Math  Operator=transpose  SaturateOnIntegerOverflow=on
  Product2 : Product  Multiplication=Matrix(*)
  Switch : Switch  Criteria=u2 > Threshold  Threshold=1
  T12_from_q12 : Subsystem
      mask help: Transforms a quaternion into a Direction Cosine Matrix
      mask Help:
      | Name:
      | 
      |     T12_from_q12
      | 
      | Description:
      | 
      |     This block implements the transformation of a quaternion into the
      |     corresponding direction cosine matrix DCM.
      | 
      | Inputs  [size] [data type] [unit]:
      | 
      |     quaternion q12 [4] [double] [-]
      | 
      | Outputs  [size] [data type] [unit]:
      | 
      |     direction cosine matrix T12  [3x3] [double] [-]
      mask Display:
      | %port_label('input', 1, 'q12')
      | %port_label('output', 1, 'T12')
      | disp('q \rightarrow DCM','texmode','on')
  rb_eom_6dof : Subsystem
  rb_eom : Outport
  wires:
  Integration/1(eom) -> rb_eom/1, Bus Selector/1
  rb_eom_6dof/3(d_qIB) -> Integration/3(d_qIB)  "d_qIB"
  rb_eom_6dof/2(d_vBII) -> Integration/2(d_vBII)  "d_vBII"
  rb_eom_6dof/1(d_pBII) -> Integration/1(d_pBII)  "d_pBII"
  Bus Selector/3 -> rb_eom_6dof/8(wBIB)  "<wBIB>"
  Bus Selector/1 -> T12_from_q12/1(q12), rb_eom_6dof/6(qIB)  "<qIB>"
  x0/1 -> Integration/5(x0)
  Bus Selector/2 -> rb_eom_6dof/7(vBII)  "<vBII>"
  T12_from_q12/1(T12) -> Math Function2/1
  Math Function2/1 -> Product2/1
  FBTX/1 -> Switch/1, Product2/2
  Product2/1 -> Switch/3
  Constant/1 -> Switch/2
  Switch/1 -> rb_eom_6dof/1(FBTB)
  MBTB/1 -> rb_eom_6dof/4(MBTB)
  mB/1 -> rb_eom_6dof/2(mB)
  d_JBB/1 -> rb_eom_6dof/5(d_JBB)
  JBB/1 -> rb_eom_6dof/3(JBB)
  rb_eom_6dof/4(d_wBIB) -> Integration/4(d_wBIB)  "d_wBIB"

== system GRM_Airframe/GRM_Airframe/stream_flow/calc_stream_flow/Subsystem1 ==
  vWEB : Inport
  vBEB : Inport  Port=2
  wBIB : Inport  Port=3
  rho : Inport  Port=4
  sos : Inport  Port=5
  AoA_Sideslip_Alphatot_Phi : Subsystem
      mask help:
      | Aus den Komponenten der Geschwindigkeit im ECEF-System, dargestellt im Body-System vBEB
      | werden Anstellwinkel (alpha), Schiebewinkel (beta), totaler Anstellwinkel (alpha_T) sowie Rollwinkel (phi) berechnet.
      | Die Ausgabe erfolgt als Bus in [rad]
      mask Help:
      | Name:
      | 
      |    AoA_sideslip_alphatot_phi
      | 
      | Beschreibung:
      | 
      |   Dieser Block berechnet Anstellwinkel, Schiebewinkel, totalen Anstellwinkel und Rollwinkel in [rad]
      |   aus der Geschwindigkeit vBEB (ECEF-System dargestellt in Body-Koordinaten)
      | 
      | Inputs   [dimension]  [data type] [unit]:
      | 
      |     vBEB    [3] [double] [m/s]
      | 
      | Outputs  [dimension]  [data type] [unit]:
      | 
      | aero_angle_bus [4] [bus] [-]
      |     alpha     [1] [double] [rad]
      |     beta       [1] [double] [rad]
      |     alpha_T [1] [double] [rad]
      |     phi         [1] [double] [rad]
      mask Display:
      | %port_label('input', 1, 'vBEB')
      | %port_label('output', 1, 'aero_angles')
      | disp('vBEB \rightarrow \alpha \beta \alpha_T \phi','texmode','on')
  Bus Selector : BusSelector  OutputSignals=al,be,th,fi
  Constant : Constant  Value=0.5
  Divide : Product  Inputs=*/
  Math Function1 : Math  Operator=square  SaturateOnIntegerOverflow=on
  Product1 : Product  Inputs=3
  Subtract : Sum  Inputs=+-
  calc_nondimensional_rates : Subsystem
  norm_of_vector : Subsystem
      mask help: computes the norm of a vector
      mask Help:
      | Name:
      | 
      |     norm_of_vector
      | 
      | Description:
      | 
      |     This block computes the L2-norm (length) of a vector.
      | 
      | Inputs  [size] [data type] [unit]:
      | 
      |     vector  [3] [double] [-]
      | 
      | Outputs  [size] [data type] [unit]:
      | 
      |     norm of vector  [1] [double] [-]
      mask Display: disp (' norm(r) ')
  al : Outport
  be : Outport  Port=2
  qdynB : Outport  Port=3
  MaB : Outport  Port=4
  a_vB : Outport  Port=5
  wBIB_star : Outport  Port=6
  th : Outport  Port=7
  fi : Outport  Port=8
  wires:
  Subtract/1 -> AoA_Sideslip_Alphatot_Phi/1(vBEB), norm_of_vector/1(vector)  "vBEB_a"
  vWEB/1 -> Subtract/2
  Bus Selector/4 -> fi/1  "<fi>"
  Bus Selector/3 -> th/1  "<th>"
  calc_nondimensional_rates/1(wBIB_star) -> wBIB_star/1
  wBIB/1 -> calc_nondimensional_rates/2(wBIB)
  Bus Selector/1 -> al/1  "<al>"
  rho/1 -> Product1/3
  Bus Selector/2 -> be/1  "<be>"
  Divide/1 -> MaB/1  "MaB"
  Constant/1 -> Product1/2
  Math Function1/1 -> Product1/1
  Product1/1 -> qdynB/1  "qdynB"
  norm_of_vector/1(norm_of_vector) -> Divide/1, a_vB/1, calc_nondimensional_rates/1(a_vB), Math Function1/1  "a_vB"
  vBEB/1 -> Subtract/1
  AoA_Sideslip_Alphatot_Phi/1(aero_angles) -> Bus Selector/1
  sos/1 -> Divide/2

== system GRM_Airframe/GRM_Airframe/stream_flow/calc_stream_flow/velocity_vector_transformation ==
  wIEE : Inport
  TIE : Inport  Port=2
  vBII : Inport  Port=3
  pBII : Inport  Port=4
  Add : Sum  Inputs=+-
  Product : Product  Multiplication=Matrix(*)
  cross_product : Subsystem
      mask help: cross product r3 = r1 x r2
      mask Help:
      | Name:
      | 
      |     cross_product
      | 
      | Description:
      | 
      |     This block implements the cross product r3 = r1 x r2.
      | 
      | Inputs  [size] [data type] [unit]:
      | 
      |     vector 1  [3] [double] [-]
      |     vector 2  [3] [double] [-]
      | 
      | Outputs  [size] [data type] [unit]:
      | 
      |     resulting vector  [3] [double] [-]
      mask Display: disp(' r3 = r1 x r2')
  vBEI : Outport
  wires:
  Add/1 -> vBEI/1  "vBEI"
  vBII/1 -> Add/1
  cross_product/1(r1_x_r2) -> Add/2  "de_vBEI"
  pBII/1 -> cross_product/2(r2)
  Product/1 -> cross_product/1(r1)  "wIEI"
  wIEE/1 -> Product/2
  TIE/1 -> Product/1

== system GRM_Airframe/GRM_Airframe/weight_and_balance/d_moi/vector2diagonal_matrix ==
  vector : Inport
  Constant6 : Constant  Value=0
  Demux : Demux  Outputs=3
  Vector Concatenate1 : Concatenate  NumInputs=3
  Vector Concatenate2 : Concatenate  NumInputs=3
  Vector Concatenate3 : Concatenate  NumInputs=3
  Vector Concatenate4 : Concatenate  NumInputs=3  Mode=Multidimensional array  ConcatenateDimension=2
  diagonal_matrix : Outport
  wires:
  Demux/3 -> Vector Concatenate3/3
  Vector Concatenate3/1 -> Vector Concatenate4/3
  Vector Concatenate1/1 -> Vector Concatenate4/1
  Vector Concatenate2/1 -> Vector Concatenate4/2
  Demux/2 -> Vector Concatenate2/2
  Vector Concatenate4/1 -> diagonal_matrix/1
  Constant6/1 -> Vector Concatenate1/2, Vector Concatenate1/3, Vector Concatenate2/1, Vector Concatenate2/3, Vector Concatenate3/1, Vector Concatenate3/2
  vector/1 -> Demux/1
  Demux/1 -> Vector Concatenate1/1

== system GRM_Airframe/GRM_Airframe/weight_and_balance/moi/JMMM_linear_interpolation ==
  mM : Inport
  Constant16 : Constant  Value=JMMM_0
  Constant17 : Constant  Value=JMMM_e
  Constant18 : Constant  Value=mM_0
  Constant19 : Constant  Value=mM_e
  Constant20 : Constant  Value=mM_0
  Constant21 : Constant  Value=JMMM_0
  Divide : Product  Inputs=**/
  Subtract : Sum  Inputs=+-
  Subtract4 : Sum  Inputs=+-
  Subtract5 : Sum  Inputs=+-
  Subtract6 : Sum
  JMMM : Outport
  wires:
  Divide/1 -> Subtract6/2
  Constant21/1 -> Subtract6/1
  Subtract6/1 -> JMMM/1  "JMMM"
  Subtract4/1 -> Divide/3
  Subtract/1 -> Divide/2
  Constant16/1 -> Subtract/2
  Constant17/1 -> Subtract/1
  Constant18/1 -> Subtract4/2
  Constant19/1 -> Subtract4/1
  Constant20/1 -> Subtract5/2
  Subtract5/1 -> Divide/1
  mM/1 -> Subtract5/1

== system GRM_Airframe/GRM_Airframe/weight_and_balance/moi/moi_coordinate_transformation ==
  JMMM : Inport
  3_rot_mat : Subsystem  mask(Rotation um 1, 2 oder 3 Achsen){rot_1=Rotation um z-Achse, rot_2=Rotation um y-Achse, rot_3=Rotation um x-Achse}
      mask prompts: rot_1 "1. Rotation"; rot_2 "2. Rotation"; rot_3 "3. Rotation"
      mask help:
      | Dieser Block liefert die Rotationsmatrix T12 für den Fall zurück, dass sich das Ziel-Koordinatensystem (1) durch Drehungen um 1, 2 oder 3 Achsen gegenüber dem Ausgangskoordinatensystem (2) beschreiben lässt (passive Drehung).
      |
      | Die Anzahl der Rotation sowie die Reihenfolge ist frei einstellbar.
      |
      | Die Rotationswinkel haben die Einheit [rad].
      mask TypeOptions rot_1: Rotation um x-Achse | Rotation um y-Achse | Rotation um z-Achse
      mask TypeOptions rot_2: Rotation um x-Achse | Rotation um y-Achse | Rotation um z-Achse
      mask TypeOptions rot_3: Rotation um x-Achse | Rotation um y-Achse | Rotation um z-Achse
  Math Function : Math  Operator=transpose  SaturateOnIntegerOverflow=on
  Matrix Multiply : Product  Multiplication=Matrix(*)
  Matrix Multiply1 : Product  Multiplication=Matrix(*)
  Thrust_rot_z : Constant  Value=unc_prp_z
  thrust_rot_x : Constant  Value=unc_prp_x
  thrust_rot_y : Constant  Value=unc_prp_y
  JMMB : Outport
  wires:
  Thrust_rot_z/1 -> 3_rot_mat/1(wi1)
  thrust_rot_x/1 -> 3_rot_mat/3(wi3)
  thrust_rot_y/1 -> 3_rot_mat/2(wi2)
  Matrix Multiply1/1 -> JMMB/1  "JMMB"
  3_rot_mat/1(T12) -> Matrix Multiply/1, Math Function/1
  JMMM/1 -> Matrix Multiply/2
  Matrix Multiply/1 -> Matrix Multiply1/1
  Math Function/1 -> Matrix Multiply1/2

== system GRM_Airframe/GRM_Airframe/weight_and_balance/moi/moi_uncertainty ==
  JBBB_c : Inport
  Add7 : Sum
  Constant16 : Constant  Value=[unc_moi_Jxx,0,0;0,unc_moi_Jyy,0;0,0,unc_moi_Jzz]
  JBBB : Outport
  wires:
  Constant16/1 -> Add7/2
  JBBB_c/1 -> Add7/1
  Add7/1 -> JBBB/1  "JBBB"

== system GRM_Airframe/GRM_Airframe/weight_and_balance/moi/steiners_theorem_missile ==
  pBPB : Inport
  Constant : Constant  Value=mB_0
  Constant17 : Constant  Value=p0PB
  Product : Product
  Subtract : Sum  Inputs=+-
  create_deviation_matrix : Subsystem
  J_deviation : Outport
  wires:
  Constant/1 -> Product/1
  Subtract/1 -> create_deviation_matrix/1(pBXB)  "pB0B"
  Constant17/1 -> Subtract/2
  create_deviation_matrix/1(T_deviation) -> Product/2
  Product/1 -> J_deviation/1
  pBPB/1 -> Subtract/1

== system GRM_Airframe/GRM_Airframe/weight_and_balance/moi/steiners_theorem_motor ==
  pBPB : Inport
  mM : Inport  Port=2
  Constant16 : Constant  Value=pMPB
  Product : Product
  Subtract4 : Sum  Inputs=+-
  create_deviation_matrix1 : Subsystem
  JM_deviation : Outport
  wires:
  mM/1 -> Product/2
  Subtract4/1 -> create_deviation_matrix1/1(pBXB)  "pBMB"
  Constant16/1 -> Subtract4/2
  create_deviation_matrix1/1(T_deviation) -> Product/1
  pBPB/1 -> Subtract4/1
  Product/1 -> JM_deviation/1

== system GRM_Airframe/GRM_Airframe/aerodynamics/aerodynamic_via_lookup/calc_aero_for_mom/cross_product ==
  note: Inputs [size]:
      |
      | r1 [3x1]
      | r2 [3x1]
  note: Outputs [size]:
      |
      | r1 x r2  [3x1]
  r1 : Inport
  r2 : Inport  Port=2
  Demux2 : Demux  Outputs=[1;1;1]
  Demux3 : Demux  Outputs=[1;1;1]
  Product{2..7} (6 alike) : Product  SaturateOnIntegerOverflow=on  RndMeth=Zero  InputSameDT=on  OutDataTypeStr=Inherit: Same as first input
  Sum : Sum  Inputs=+-  SaturateOnIntegerOverflow=on  InputSameDT=on  OutDataTypeStr=Inherit: Same as first input
  Sum1 : Sum  Inputs=+-  SaturateOnIntegerOverflow=on  InputSameDT=on  OutDataTypeStr=Inherit: Same as first input
  Sum2 : Sum  Inputs=+-  SaturateOnIntegerOverflow=on  InputSameDT=on  OutDataTypeStr=Inherit: Same as first input
  Vector Concatenate : Concatenate  NumInputs=3  Mode=Multidimensional array
  r1_x_r2 : Outport  PortDimensions=[3,1]
  wires:
  Vector Concatenate/1 -> r1_x_r2/1
  r2/1 -> Demux3/1
  r1/1 -> Demux2/1
  Sum2/1 -> Vector Concatenate/3
  Sum1/1 -> Vector Concatenate/2
  Sum/1 -> Vector Concatenate/1
  Product7/1 -> Sum2/2
  Product6/1 -> Sum2/1
  Product5/1 -> Sum1/2
  Product4/1 -> Sum1/1
  Product3/1 -> Sum/2
  Product2/1 -> Sum/1
  Demux2/1 -> Product5/1, Product6/1
  Demux3/1 -> Product4/2, Product7/2
  Demux2/3 -> Product4/1, Product3/1
  Demux3/2 -> Product3/2, Product6/2
  Demux3/3 -> Product2/2, Product5/2
  Demux2/2 -> Product7/1, Product2/1
